simulink model "parallel_min_cost_function_vopt_6phase"  (R2022a)
settings: Solver=FixedStepDiscrete  StartTime=0.0  StopTime=10.0  RelTol=1e-3
undefined symbols (not defined in the file or in its folder): f_c
libraries: hdlsllib x18
settings Model: DataTypeOverride=Off  Creator=Andre Merx  LastModifiedBy=Andre Merx
settings SolverCC: AlgebraicLoopSolver=TrustRegion
settings DataIOCC: LimitDataPoints=on  SaveOutput=off  SaveTime=off
settings OptimizationCC: BlockReduction=off  ConditionallyExecuteInputs=off  DefaultParameterBehavior=Inlined  LifeSpan=inf
settings DebuggingCC: AlgebraicLoopMsg=error  SingleTaskRateTransMsg=error  UnconnectedInputMsg=warning  UnconnectedOutputMsg=warning  UnconnectedLineMsg=warning  AllowSymbolicDim=off  StrictBusMsg=ErrorOnBusTreatedAsVector  SFUnexpectedBacktrackingDiag=warning  SFNoUnconditionalDefaultTransitionDiag=warning  SFExecutionAtInitializationDiag=none  SFMachineParentedDataDiag=warning  ArithmeticOperatorsInVariantConditions=warning
settings HardwareCC: ProdBitPerPointer=32  ProdBitPerSizeT=32  ProdBitPerPtrDiffT=32  ProdLargestAtomicFloat=None  ProdIntDivRoundTo=Undefined  ProdEndianess=Unspecified  ProdWordSize=32  ProdHWDeviceType=ASIC/FPGA->ASIC/FPGA  ProdEqTarget=off
settings SFSimCC: SimUseLocalCustomCode=off  CustomCodeUndefinedFunction=UseInterfaceOnly
settings RTWCC: RTWUseLocalCustomCode=off
settings CodeAppCC: StateflowObjectComments=on
settings GRTTargetCC: TargetLangStandard=C89/C90 (ANSI)
settings ConfigComp: CovScope=ReferencedModels  CovMetricSettings=dw  CovSaveCumulativeToWorkspaceVar=on  CovSaveSingleToWorkspaceVar=on  CovExternalEMLEnable=off  CovSFcnEnable=off

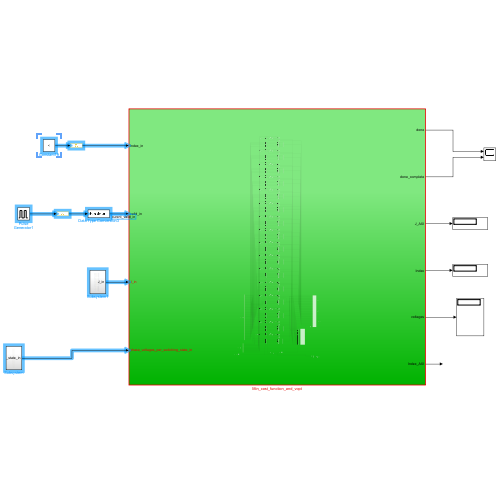
[thumbnail: Simulink's stored preview of the top-level diagram]
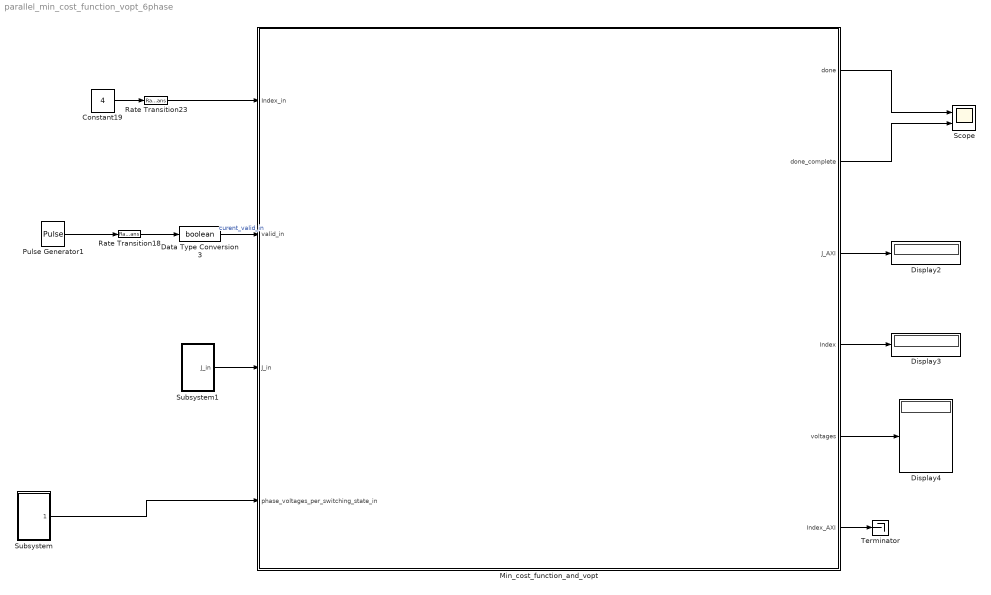
== system parallel_min_cost_function_vopt_6phase ==
  Constant19 : Constant  Value=4  OutDataTypeStr=int32  SampleTime=-1
  Data Type Conversion3 : DataTypeConversion  OutDataTypeStr=boolean  SaturateOnIntegerOverflow=off  RndMeth=Floor
  Display2 : Display
  Display3 : Display
  Display4 : Display
  Min_cost_function_and_vopt : Subsystem  TreatAsAtomicUnit=on
  Pulse Generator1 : DiscretePulseGenerator  PulseType=Time based  Period=1/f_c
  Rate Transition18 : RateTransition  OutPortSampleTime=Rt
  Rate Transition23 : RateTransition  OutPortSampleTime=Rt
  Scope : Scope  NumInputPorts=2
  Subsystem : Subsystem
  Subsystem1 : Subsystem
  Terminator : Terminator
  wires:
  Rate Transition23/1 -> Min_cost_function_and_vopt/1(Index_in)
  Constant19/1 -> Rate Transition23/1
  Rate Transition18/1 -> Data Type Conversion3/1
  Data Type Conversion3/1 -> Min_cost_function_and_vopt/2(valid_in)  "curent_valid_in"
  Pulse Generator1/1 -> Rate Transition18/1
  Subsystem1/1(J_in) -> Min_cost_function_and_vopt/3(J_in)
  Subsystem/1(phase_voltages_per_switching_state_in) -> Min_cost_function_and_vopt/4(phase_voltages_per_switching_state_in)
  Min_cost_function_and_vopt/1(done) -> Scope/1
  Min_cost_function_and_vopt/2(done_complete) -> Scope/2
  Min_cost_function_and_vopt/3(J_AXI) -> Display2/1
  Min_cost_function_and_vopt/4(Index) -> Display3/1
  Min_cost_function_and_vopt/5(voltages) -> Display4/1
  Min_cost_function_and_vopt/6(Index_AXI) -> Terminator/1

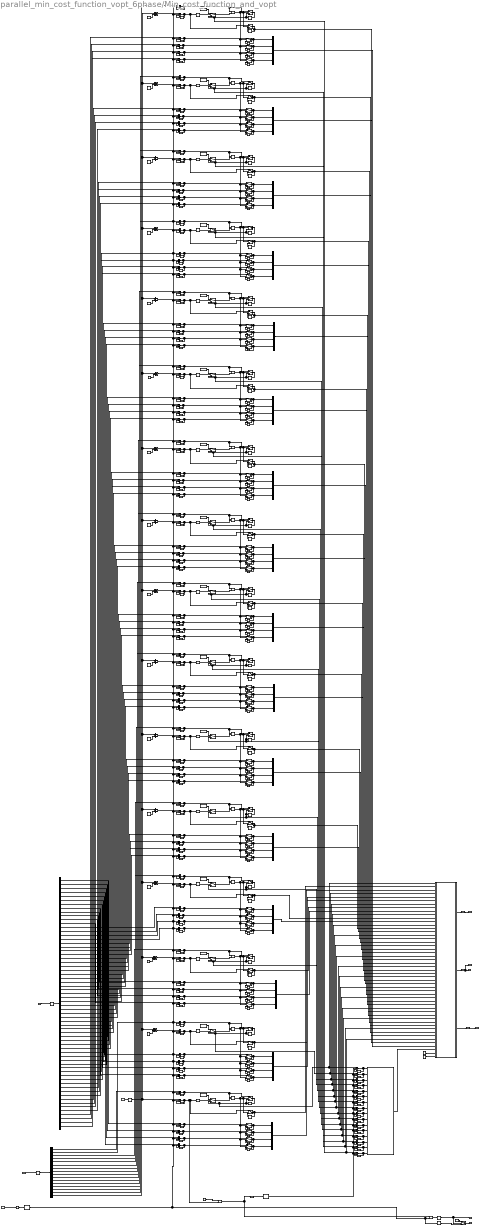
== system parallel_min_cost_function_vopt_6phase/Min_cost_function_and_vopt ==
  Index_in : Inport
  valid_in : Inport  Port=2
  J_in : Inport  Port=3
  phase_voltages_per_switching_state_in : Inport  Port=4
  Add{,1..14} (15 alike) : Sum
  Compare To Constant : hdlsllib/Logic and Bit Operations/Compare To Constant  relop=<=  const=1  OutDataTypeStr=boolean
      settings: SourceProductBaseCode=SL
  Compare To Constant1 : hdlsllib/Logic and Bit Operations/Compare To Constant  relop=<=  const=5  OutDataTypeStr=boolean
      settings: SourceProductBaseCode=SL
  Compare To Constant10 : hdlsllib/Logic and Bit Operations/Compare To Constant  relop=<=  const=41  OutDataTypeStr=boolean
      settings: SourceProductBaseCode=SL
  Compare To Constant11 : hdlsllib/Logic and Bit Operations/Compare To Constant  relop=<=  const=45  OutDataTypeStr=boolean
      settings: SourceProductBaseCode=SL
  Compare To Constant12 : hdlsllib/Logic and Bit Operations/Compare To Constant  relop=<=  const=49  OutDataTypeStr=boolean
      settings: SourceProductBaseCode=SL
  Compare To Constant13 : hdlsllib/Logic and Bit Operations/Compare To Constant  relop=<=  const=53  OutDataTypeStr=boolean
      settings: SourceProductBaseCode=SL
  Compare To Constant14 : hdlsllib/Logic and Bit Operations/Compare To Constant  relop=<=  const=57  OutDataTypeStr=boolean
      settings: SourceProductBaseCode=SL
  Compare To Constant15 : hdlsllib/Logic and Bit Operations/Compare To Constant  relop=<=  const=61  OutDataTypeStr=boolean
      settings: SourceProductBaseCode=SL
  Compare To Constant2 : hdlsllib/Logic and Bit Operations/Compare To Constant  relop=<=  const=9  OutDataTypeStr=boolean
      settings: SourceProductBaseCode=SL
  Compare To Constant3 : hdlsllib/Logic and Bit Operations/Compare To Constant  relop=<=  const=13  OutDataTypeStr=boolean
      settings: SourceProductBaseCode=SL
  Compare To Constant4 : hdlsllib/Logic and Bit Operations/Compare To Constant  relop=<=  const=17  OutDataTypeStr=boolean
      settings: SourceProductBaseCode=SL
  Compare To Constant5 : hdlsllib/Logic and Bit Operations/Compare To Constant  relop=<=  const=21  OutDataTypeStr=boolean
      settings: SourceProductBaseCode=SL
  Compare To Constant6 : hdlsllib/Logic and Bit Operations/Compare To Constant  relop=<=  const=25  OutDataTypeStr=boolean
      settings: SourceProductBaseCode=SL
  Compare To Constant7 : hdlsllib/Logic and Bit Operations/Compare To Constant  relop=<=  const=29  OutDataTypeStr=boolean
      settings: SourceProductBaseCode=SL
  Compare To Constant8 : hdlsllib/Logic and Bit Operations/Compare To Constant  relop=<=  const=33  OutDataTypeStr=boolean
      settings: SourceProductBaseCode=SL
  Compare To Constant9 : hdlsllib/Logic and Bit Operations/Compare To Constant  relop=<=  const=37  OutDataTypeStr=boolean
      settings: SourceProductBaseCode=SL
  Constant{,3..17} (16 alike) : Constant  Value=250  OutDataTypeStr=fixdt(1,20,11)  SampleTime=-1
  Constant1 : Constant  Value=4  OutDataTypeStr=int32  SampleTime=-1
  Constant18 : Constant  Value=4  OutDataTypeStr=int32  SampleTime=-1
  Constant19 : Constant  Value=8  OutDataTypeStr=int32  SampleTime=-1
  Constant2 : Constant  Value=0  OutDataTypeStr=boolean  SampleTime=-1
  Constant20 : Constant  Value=12  OutDataTypeStr=int32  SampleTime=-1
  Constant21 : Constant  Value=16  OutDataTypeStr=int32  SampleTime=-1
  Constant22 : Constant  Value=20  OutDataTypeStr=int32  SampleTime=-1
  Constant23 : Constant  Value=24  OutDataTypeStr=int32  SampleTime=-1
  Constant24 : Constant  Value=28  OutDataTypeStr=int32  SampleTime=-1
  Constant25 : Constant  Value=32  OutDataTypeStr=int32  SampleTime=-1
  Constant26 : Constant  Value=36  OutDataTypeStr=int32  SampleTime=-1
  Constant27 : Constant  Value=40  OutDataTypeStr=int32  SampleTime=-1
  Constant28 : Constant  Value=44  OutDataTypeStr=int32  SampleTime=-1
  Constant29 : Constant  Value=48  OutDataTypeStr=int32  SampleTime=-1
  Constant30 : Constant  Value=52  OutDataTypeStr=int32  SampleTime=-1
  Constant31 : Constant  Value=56  OutDataTypeStr=int32  SampleTime=-1
  Constant32 : Constant  Value=60  OutDataTypeStr=int32  SampleTime=-1
  Constant33 : Constant  Value=0  OutDataTypeStr=fixdt(1,20,11)  SampleTime=-1
  Constant34 : Constant  Value=[0;0;0;0]  OutDataTypeStr=fixdt(1,24,11)  SampleTime=-1
  Delay{,1..5,7..8,12..22,25..26,34..43,46,49..50,58..67,72..73,81..90,95..96,104..113,118..119,127..136,141..142,150..159,164..165,173..182,191..200,205..206,214..223,228..229,237..246,251..252,260..269,274..275,283..292,297..298,302..303,311..320,325..326,334..343,348..349,357..366,371..386} (216 alike) : Delay  DelayLength=1
  Delay23 : Delay  DelayLength=3
  Delay24 : Delay  DelayLength=3
  Demux : Demux  Outputs=16
  Demux1 : Demux  Outputs=64
  Detect Rise Positive : hdlsllib/Logic and Bit Operations/Detect Rise Positive  vinit=0  OutDataTypeStr=boolean
      settings: SourceProductBaseCode=SL
  Detect Rise Positive1 : hdlsllib/Logic and Bit Operations/Detect Rise Positive  vinit=0  OutDataTypeStr=boolean
      settings: SourceProductBaseCode=SL
  Logical Operator : Logic  AllPortsSameDT=off  OutDataTypeStr=boolean
  MATLAB Function : MATLAB Function  TreatAsAtomicUnit=on
  MinMax : MinMax  Inputs=16
  Mux{,1..15} (16 alike) : Mux
  Relational Operator{,2..16} (16 alike) : RelationalOperator  Operator=<=  OutDataTypeStr=boolean  RndMeth=Simplest  InputSameDT=off
  Relational Operator1 : RelationalOperator  Operator===  OutDataTypeStr=boolean  RndMeth=Simplest  InputSameDT=off
  Switch{,1,8..9,20..21,27..28,34..35,41..42,48..49,55..56,62..63,69..70,76..77,83..84,90..91,97..98,104..105,111..112} (32 alike) : Switch  Criteria=u2 > Threshold  OutDataTypeStr=fixdt(1,20,11)  SaturateOnIntegerOverflow=off  InputSameDT=off
  Switch{2,10,15,22,29,36,43,50,57,64,71,78,85,92,99,106} (16 alike) : Switch  Criteria=u2 > Threshold  OutDataTypeStr=int32  SaturateOnIntegerOverflow=off  InputSameDT=off
  Switch{3..6,11..14,16..19,23..26,30..33,37..40,44..47,51..54,58..61,65..68,72..75,79..82,86..89,93..96,100..103,107..110} (64 alike) : Switch  Criteria=u2 > Threshold  OutDataTypeStr=fixdt(1,24,11)  SaturateOnIntegerOverflow=off  InputSameDT=off
  Switch7 : Switch  Criteria=u2 > Threshold  SaturateOnIntegerOverflow=off  InputSameDT=off
  Switch_on{1,4,7,10,14,17,20,23,26,29,32,35,38,41,44,47,50,53,56,59,62,65,68,71,74,77,80,83,86,89,92,95,98..113} (48 alike) : Switch  Threshold=1  OutDataTypeStr=Inherit: Inherit via back propagation  RndMeth=Simplest  SaturateOnIntegerOverflow=off  InputSameDT=off
  Switch_on{2..3,5..6,8..9,11..12,15..16,18..19,21..22,24..25,27..28,30..31,33..34,36..37,39..40,42..43,45..46,48..49,51..52,54..55,57..58,60..61,63..64,66..67,69..70,72..73,75..76,78..79,81..82,84..85,87..88,90..91,93..94,96..97} (64 alike) : Switch  Threshold=1  OutDataTypeStr=fixdt(1,24,11)  RndMeth=Simplest  SaturateOnIntegerOverflow=off  InputSameDT=off
      Switch_on49 settings: LockScale=on
  done : Outport
  done_complete : Outport  Port=2
  J_AXI : Outport  Port=3
  Index : Outport  Port=4
  voltages : Outport  Port=5
  Index_AXI : Outport  Port=6
  wires:
  Demux/1 -> Switch_on4/1  "End_Cycle"
  Demux1/1 -> Switch_on2/1  "End_Cycle"
  Demux1/2 -> Switch_on3/1  "End_Cycle"
  Switch5/1 -> Mux/3, Delay4/1
  Delay3/1 -> Switch4/3
  Relational Operator/1 -> Switch5/2, Switch6/2, Switch4/2, Switch3/2, Switch2/2, Switch1/2
  Compare To Constant/1 -> Switch/2
  Switch1/1 -> Delay/1
  Switch6/1 -> Delay5/1, Mux/4
  Delay4/1 -> Switch5/3
  Switch4/1 -> Mux/2, Delay3/1
  Switch/1 -> Relational Operator/2
  Delay1/1 -> Switch2/3
  Delay5/1 -> Switch6/3
  Switch3/1 -> Mux/1, Delay2/1
  Delay2/1 -> Switch3/3
  Constant/1 -> Switch/1
  Switch_on4/1 -> Relational Operator/1, Switch1/1, Delay17/1
  Switch_on1/1 -> Delay18/1, Relational Operator1/2, Switch2/1, Compare To Constant/1
  Switch_on2/1 -> Delay19/1, Switch3/1
  Switch_on3/1 -> Delay20/1, Switch4/1
  Switch_on5/1 -> Switch5/1, Delay21/1
  Switch_on6/1 -> Switch6/1, Delay22/1
  Delay46/1 -> Detect Rise Positive/1
  valid_in/1 -> Delay46/1  "End_Cycle"
  Delay17/1 -> Switch_on4/3
  Delay8/1 -> Switch_on1/1, Add/1, Add3/1, Add7/1, Add10/1, Add12/1, Add14/1, Add13/1, Add11/1, Add9/1, Add8/1, Add6/1, Add5/1, Add4/1, Add2/1, Add1/1
  Delay18/1 -> Switch_on1/3
  Delay19/1 -> Switch_on2/3
  Delay20/1 -> Switch_on3/3
  Delay21/1 -> Switch_on5/3
  Delay22/1 -> Switch_on6/3
  Delay23/1 -> Switch7/2, done_complete/1
  Logical Operator/1 -> Delay23/1
  Delay24/1 -> Switch7/3
  Constant1/1 -> Relational Operator1/1
  Constant2/1 -> Switch7/1
  Switch7/1 -> done/1
  Demux1/3 -> Switch_on5/1  "End_Cycle"
  Demux1/4 -> Switch_on6/1  "End_Cycle"
  Demux/2 -> Switch_on10/1  "End_Cycle"
  Delay34/1 -> Switch_on10/3
  Switch8/1 -> Relational Operator2/2
  Switch_on8/1 -> Delay36/1, Switch11/1
  Demux1/6 -> Switch_on9/1  "End_Cycle"
  Delay26/1 -> Switch10/3
  Add/1 -> Switch_on7/1
  Delay36/1 -> Switch_on8/3
  Delay39/1 -> Switch_on11/3
  Switch_on7/1 -> Delay35/1, Switch10/1, Compare To Constant1/1
  Compare To Constant1/1 -> Switch8/2
  Switch_on9/1 -> Delay38/1, Switch12/1
  Delay40/1 -> Switch_on12/3
  Delay35/1 -> Switch_on7/3
  Switch_on11/1 -> Switch13/1, Delay39/1
  Delay43/1 -> Switch14/3
  Switch_on12/1 -> Switch14/1, Delay40/1
  Delay37/1 -> Switch11/3
  Relational Operator2/1 -> Switch13/2, Switch14/2, Switch12/2, Switch11/2, Switch10/2, Switch9/2
  Switch9/1 -> Delay25/1
  Delay42/1 -> Switch13/3
  Demux1/5 -> Switch_on8/1  "End_Cycle"
  Demux1/7 -> Switch_on11/1  "End_Cycle"
  Switch_on10/1 -> Relational Operator2/1, Switch9/1, Delay34/1
  Demux1/8 -> Switch_on12/1  "End_Cycle"
  Delay38/1 -> Switch_on9/3
  Constant3/1 -> Switch8/1
  Delay41/1 -> Switch12/3
  Delay61/1 -> Switch16/3
  Switch_on16/1 -> Switch19/1, Delay64/1
  Delay67/1 -> Switch19/3
  Switch_on15/1 -> Switch18/1, Delay63/1
  Delay59/1 -> Switch_on17/3
  Switch_on19/1 -> Delay62/1, Switch17/1
  Delay64/1 -> Switch_on16/3
  Switch_on17/1 -> Delay59/1, Switch15/1, Compare To Constant2/1
  Compare To Constant2/1 -> Switch20/2
  Demux1/10 -> Switch_on19/1  "End_Cycle"
  Delay50/1 -> Switch15/3
  Switch20/1 -> Relational Operator3/2
  Demux/3 -> Switch_on14/1  "End_Cycle"
  Delay65/1 -> Switch17/3
  Switch_on14/1 -> Relational Operator3/1, Switch21/1, Delay58/1
  Switch_on18/1 -> Delay60/1, Switch16/1
  Constant4/1 -> Switch20/1
  Demux1/11 -> Switch_on15/1  "End_Cycle"
  Delay63/1 -> Switch_on15/3
  Delay66/1 -> Switch18/3
  Switch21/1 -> Delay49/1
  Demux1/9 -> Switch_on18/1  "End_Cycle"
  Demux1/12 -> Switch_on16/1  "End_Cycle"
  Add1/1 -> Switch_on17/1
  Delay60/1 -> Switch_on18/3
  Relational Operator3/1 -> Switch18/2, Switch19/2, Switch17/2, Switch16/2, Switch15/2, Switch21/2
  Delay58/1 -> Switch_on14/3
  Delay62/1 -> Switch_on19/3
  Delay84/1 -> Switch23/3
  Switch_on22/1 -> Switch26/1, Delay87/1
  Delay90/1 -> Switch26/3
  Switch_on21/1 -> Switch25/1, Delay86/1
  Delay82/1 -> Switch_on23/3
  Switch_on25/1 -> Delay85/1, Switch24/1
  Delay87/1 -> Switch_on22/3
  Switch_on23/1 -> Delay82/1, Switch22/1, Compare To Constant3/1
  Compare To Constant3/1 -> Switch27/2
  Demux1/14 -> Switch_on25/1  "End_Cycle"
  Delay73/1 -> Switch22/3
  Switch27/1 -> Relational Operator4/2
  Demux/4 -> Switch_on20/1  "End_Cycle"
  Delay88/1 -> Switch24/3
  Switch_on20/1 -> Relational Operator4/1, Switch28/1, Delay81/1
  Switch_on24/1 -> Delay83/1, Switch23/1
  Constant5/1 -> Switch27/1
  Demux1/15 -> Switch_on21/1  "End_Cycle"
  Delay86/1 -> Switch_on21/3
  Delay89/1 -> Switch25/3
  Switch28/1 -> Delay72/1
  Demux1/13 -> Switch_on24/1  "End_Cycle"
  Demux1/16 -> Switch_on22/1  "End_Cycle"
  Add2/1 -> Switch_on23/1
  Delay83/1 -> Switch_on24/3
  Relational Operator4/1 -> Switch25/2, Switch26/2, Switch24/2, Switch23/2, Switch22/2, Switch28/2
  Delay81/1 -> Switch_on20/3
  Delay85/1 -> Switch_on25/3
  Delay107/1 -> Switch30/3
  Switch_on28/1 -> Switch33/1, Delay110/1
  Delay113/1 -> Switch33/3
  Switch_on27/1 -> Switch32/1, Delay109/1
  Delay105/1 -> Switch_on29/3
  Switch_on31/1 -> Delay108/1, Switch31/1
  Delay110/1 -> Switch_on28/3
  Switch_on29/1 -> Delay105/1, Switch29/1, Compare To Constant4/1
  Compare To Constant4/1 -> Switch34/2
  Demux1/18 -> Switch_on31/1  "End_Cycle"
  Delay96/1 -> Switch29/3
  Switch34/1 -> Relational Operator5/2
  Demux/5 -> Switch_on26/1  "End_Cycle"
  Delay111/1 -> Switch31/3
  Switch_on26/1 -> Relational Operator5/1, Switch35/1, Delay104/1
  Switch_on30/1 -> Delay106/1, Switch30/1
  Constant6/1 -> Switch34/1
  Demux1/19 -> Switch_on27/1  "End_Cycle"
  Delay109/1 -> Switch_on27/3
  Delay112/1 -> Switch32/3
  Switch35/1 -> Delay95/1
  Demux1/17 -> Switch_on30/1  "End_Cycle"
  Demux1/20 -> Switch_on28/1  "End_Cycle"
  Add3/1 -> Switch_on29/1
  Delay106/1 -> Switch_on30/3
  Relational Operator5/1 -> Switch32/2, Switch33/2, Switch31/2, Switch30/2, Switch29/2, Switch35/2
  Delay104/1 -> Switch_on26/3
  Delay108/1 -> Switch_on31/3
  Delay130/1 -> Switch37/3
  Switch_on34/1 -> Switch40/1, Delay133/1
  Delay136/1 -> Switch40/3
  Switch_on33/1 -> Switch39/1, Delay132/1
  Delay128/1 -> Switch_on35/3
  Switch_on37/1 -> Delay131/1, Switch38/1
  Delay133/1 -> Switch_on34/3
  Switch_on35/1 -> Delay128/1, Switch36/1, Compare To Constant5/1
  Compare To Constant5/1 -> Switch41/2
  Demux1/22 -> Switch_on37/1  "End_Cycle"
  Delay119/1 -> Switch36/3
  Switch41/1 -> Relational Operator6/2
  Demux/6 -> Switch_on32/1  "End_Cycle"
  Delay134/1 -> Switch38/3
  Switch_on32/1 -> Relational Operator6/1, Switch42/1, Delay127/1
  Switch_on36/1 -> Delay129/1, Switch37/1
  Constant7/1 -> Switch41/1
  Demux1/23 -> Switch_on33/1  "End_Cycle"
  Delay132/1 -> Switch_on33/3
  Delay135/1 -> Switch39/3
  Switch42/1 -> Delay118/1
  Demux1/21 -> Switch_on36/1  "End_Cycle"
  Demux1/24 -> Switch_on34/1  "End_Cycle"
  Add4/1 -> Switch_on35/1
  Delay129/1 -> Switch_on36/3
  Relational Operator6/1 -> Switch39/2, Switch40/2, Switch38/2, Switch37/2, Switch36/2, Switch42/2
  Delay127/1 -> Switch_on32/3
  Delay131/1 -> Switch_on37/3
  Delay153/1 -> Switch44/3
  Switch_on40/1 -> Switch47/1, Delay156/1
  Delay159/1 -> Switch47/3
  Switch_on39/1 -> Switch46/1, Delay155/1
  Delay151/1 -> Switch_on41/3
  Switch_on43/1 -> Delay154/1, Switch45/1
  Delay156/1 -> Switch_on40/3
  Switch_on41/1 -> Delay151/1, Switch43/1, Compare To Constant6/1
  Compare To Constant6/1 -> Switch48/2
  Demux1/26 -> Switch_on43/1  "End_Cycle"
  Delay142/1 -> Switch43/3
  Switch48/1 -> Relational Operator7/2
  Delay157/1 -> Switch45/3
  Switch_on38/1 -> Relational Operator7/1, Switch49/1, Delay150/1
  Switch_on42/1 -> Delay152/1, Switch44/1
  Constant8/1 -> Switch48/1
  Demux1/27 -> Switch_on39/1  "End_Cycle"
  Delay155/1 -> Switch_on39/3
  Delay158/1 -> Switch46/3
  Switch49/1 -> Delay141/1
  Demux1/25 -> Switch_on42/1  "End_Cycle"
  Demux1/28 -> Switch_on40/1  "End_Cycle"
  Add5/1 -> Switch_on41/1
  Delay152/1 -> Switch_on42/3
  Relational Operator7/1 -> Switch46/2, Switch47/2, Switch45/2, Switch44/2, Switch43/2, Switch49/2
  Delay150/1 -> Switch_on38/3
  Delay154/1 -> Switch_on43/3
  Delay176/1 -> Switch51/3
  Switch_on46/1 -> Switch54/1, Delay179/1
  Delay182/1 -> Switch54/3
  Switch_on45/1 -> Switch53/1, Delay178/1
  Delay174/1 -> Switch_on47/3
  Switch_on49/1 -> Delay177/1, Switch52/1
  Delay179/1 -> Switch_on46/3
  Switch_on47/1 -> Delay174/1, Switch50/1, Compare To Constant7/1
  Compare To Constant7/1 -> Switch55/2
  Demux1/30 -> Switch_on49/1  "End_Cycle"
  Delay165/1 -> Switch50/3
  Switch55/1 -> Relational Operator8/2
  Demux/8 -> Switch_on44/1  "End_Cycle"
  Delay180/1 -> Switch52/3
  Switch_on44/1 -> Relational Operator8/1, Switch56/1, Delay173/1
  Switch_on48/1 -> Delay175/1, Switch51/1
  Constant9/1 -> Switch55/1
  Demux1/31 -> Switch_on45/1  "End_Cycle"
  Delay178/1 -> Switch_on45/3
  Delay181/1 -> Switch53/3
  Switch56/1 -> Delay164/1
  Demux1/29 -> Switch_on48/1  "End_Cycle"
  Demux1/32 -> Switch_on46/1  "End_Cycle"
  Add6/1 -> Switch_on47/1
  Delay175/1 -> Switch_on48/3
  Relational Operator8/1 -> Switch53/2, Switch54/2, Switch52/2, Switch51/2, Switch50/2, Switch56/2
  Delay173/1 -> Switch_on44/3
  Delay177/1 -> Switch_on49/3
  Delay264/1 -> Switch_on79/3
  Relational Operator13/1 -> Switch88/2, Switch89/2, Switch87/2, Switch86/2, Switch85/2, Switch91/2
  Add11/1 -> Switch_on77/1
  Demux1/49 -> Switch_on78/1  "End_Cycle"
  Demux1/51 -> Switch_on75/1  "End_Cycle"
  Delay268/1 -> Switch88/3
  Constant14/1 -> Switch90/1
  Delay252/1 -> Switch85/3
  Compare To Constant12/1 -> Switch90/2
  Switch_on75/1 -> Switch88/1, Delay265/1
  Delay291/1 -> Switch60/3
  Demux1/35 -> Switch_on51/1  "End_Cycle"
  Switch_on74/1 -> Relational Operator13/1, Switch91/1, Delay260/1
  Demux/13 -> Switch_on74/1  "End_Cycle"
  Switch_on54/1 -> Delay285/1, Switch58/1
  Delay290/1 -> Switch59/3
  Relational Operator9/1 -> Switch60/2, Switch61/2, Switch59/2, Switch58/2, Switch57/2, Switch63/2
  Switch90/1 -> Relational Operator13/2
  Delay285/1 -> Switch_on54/3
  Switch_on55/1 -> Delay287/1, Switch59/1
  Delay284/1 -> Switch_on53/3
  Delay292/1 -> Switch61/3
  Switch_on52/1 -> Switch61/1, Delay289/1
  Switch62/1 -> Relational Operator9/2
  Demux/9 -> Switch_on50/1  "End_Cycle"
  Demux1/34 -> Switch_on55/1  "End_Cycle"
  Compare To Constant8/1 -> Switch62/2
  Switch_on53/1 -> Delay284/1, Switch57/1, Compare To Constant8/1
  Delay192/1 -> Switch_on59/3
  Switch_on57/1 -> Switch67/1, Delay196/1
  Switch_on58/1 -> Switch68/1, Delay197/1
  Demux1/52 -> Switch_on76/1  "End_Cycle"
  Compare To Constant11/1 -> Switch83/2
  Constant10/1 -> Switch62/1
  Switch_on73/1 -> Delay241/1, Switch80/1
  Delay262/1 -> Switch_on78/3
  Switch_on69/1 -> Switch81/1, Delay242/1
  Delay246/1 -> Switch82/3
  Delay266/1 -> Switch_on76/3
  Delay263/1 -> Switch86/3
  Switch_on70/1 -> Switch82/1, Delay243/1
  Delay240/1 -> Switch79/3
  Demux1/40 -> Switch_on58/1  "End_Cycle"
  Switch70/1 -> Delay297/1
  Delay199/1 -> Switch67/3
  Delay194/1 -> Switch65/3
  Demux1/33 -> Switch_on54/1  "End_Cycle"
  Demux1/39 -> Switch_on57/1  "End_Cycle"
  Delay196/1 -> Switch_on57/3
  Constant11/1 -> Switch69/1
  Switch_on78/1 -> Delay262/1, Switch86/1
  Switch_on60/1 -> Delay193/1, Switch65/1
  Delay298/1 -> Switch64/3
  Demux/10 -> Switch_on56/1  "End_Cycle"
  Demux1/38 -> Switch_on61/1  "End_Cycle"
  Switch_on56/1 -> Relational Operator10/1, Switch70/1, Delay191/1
  Switch_on79/1 -> Delay264/1, Switch87/1
  Delay198/1 -> Switch66/3
  Demux1/50 -> Switch_on79/1  "End_Cycle"
  Delay269/1 -> Switch89/3
  Delay197/1 -> Switch_on58/3
  Switch_on59/1 -> Delay192/1, Switch64/1, Compare To Constant9/1
  Delay243/1 -> Switch_on70/3
  Delay286/1 -> Switch58/3
  Switch_on76/1 -> Switch89/1, Delay266/1
  Delay287/1 -> Switch_on55/3
  Delay289/1 -> Switch_on52/3
  Switch_on51/1 -> Switch60/1, Delay288/1
  Delay239/1 -> Switch_on72/3
  Delay275/1 -> Switch57/3
  Add10/1 -> Switch_on71/1
  Relational Operator12/1 -> Switch81/2, Switch82/2, Switch80/2, Switch79/2, Switch78/2, Switch84/2
  Demux1/48 -> Switch_on70/1  "End_Cycle"
  Demux1/45 -> Switch_on72/1  "End_Cycle"
  Switch84/1 -> Delay228/1
  Demux1/47 -> Switch_on69/1  "End_Cycle"
  Constant13/1 -> Switch83/1
  Switch_on72/1 -> Delay239/1, Switch79/1
  Delay267/1 -> Switch87/3
  Switch_on68/1 -> Relational Operator12/1, Switch84/1, Delay237/1
  Switch83/1 -> Relational Operator12/2
  Demux1/37 -> Switch_on60/1  "End_Cycle"
  Delay229/1 -> Switch78/3
  Delay195/1 -> Switch_on61/3
  Switch69/1 -> Relational Operator10/2
  Delay217/1 -> Switch72/3
  Delay265/1 -> Switch_on75/3
  Demux1/46 -> Switch_on73/1  "End_Cycle"
  Switch_on63/1 -> Switch74/1, Delay219/1
  Switch_on64/1 -> Switch75/1, Delay220/1
  Delay244/1 -> Switch80/3
  Switch_on71/1 -> Delay238/1, Switch78/1, Compare To Constant11/1
  Delay220/1 -> Switch_on64/3
  Delay223/1 -> Switch75/3
  Switch_on61/1 -> Delay195/1, Switch66/1
  Demux1/36 -> Switch_on52/1  "End_Cycle"
  Switch_on67/1 -> Delay218/1, Switch73/1
  Delay218/1 -> Switch_on67/3
  Delay193/1 -> Switch_on60/3
  Delay191/1 -> Switch_on56/3
  Switch63/1 -> Delay274/1
  Delay261/1 -> Switch_on77/3
  Relational Operator11/1 -> Switch74/2, Switch75/2, Switch73/2, Switch72/2, Switch71/2, Switch77/2
  Delay214/1 -> Switch_on62/3
  Delay242/1 -> Switch_on69/3
  Delay216/1 -> Switch_on66/3
  Add9/1 -> Switch_on65/1
  Switch77/1 -> Delay205/1
  Switch_on50/1 -> Relational Operator9/1, Switch63/1, Delay283/1
  Delay200/1 -> Switch68/3
  Delay222/1 -> Switch74/3
  Delay219/1 -> Switch_on63/3
  Delay288/1 -> Switch_on51/3
  Demux1/43 -> Switch_on63/1  "End_Cycle"
  Add8/1 -> Switch_on59/1
  Switch_on66/1 -> Delay216/1, Switch72/1
  Demux1/44 -> Switch_on64/1  "End_Cycle"
  Delay260/1 -> Switch_on74/3
  Compare To Constant9/1 -> Switch69/2
  Constant12/1 -> Switch76/1
  Delay245/1 -> Switch81/3
  Demux/11 -> Switch_on62/1  "End_Cycle"
  Delay206/1 -> Switch71/3
  Delay215/1 -> Switch_on65/3
  Delay221/1 -> Switch73/3
  Demux/12 -> Switch_on68/1  "End_Cycle"
  Add7/1 -> Switch_on53/1
  Switch76/1 -> Relational Operator11/2
  Delay241/1 -> Switch_on73/3
  Delay238/1 -> Switch_on71/3
  Relational Operator10/1 -> Switch67/2, Switch68/2, Switch66/2, Switch65/2, Switch64/2, Switch70/2
  Compare To Constant10/1 -> Switch76/2
  Switch_on65/1 -> Delay215/1, Switch71/1, Compare To Constant10/1
  Switch_on77/1 -> Delay261/1, Switch85/1, Compare To Constant12/1
  Delay283/1 -> Switch_on50/3
  Delay237/1 -> Switch_on68/3
  Demux1/41 -> Switch_on66/1  "End_Cycle"
  Switch_on62/1 -> Relational Operator11/1, Switch77/1, Delay214/1
  Demux1/42 -> Switch_on67/1  "End_Cycle"
  Switch91/1 -> Delay251/1
  Switch_on83/1 -> Delay312/1, Switch92/1, Compare To Constant13/1
  Switch112/1 -> Delay348/1
  Compare To Constant13/1 -> Switch97/2
  Delay335/1 -> Switch_on89/3
  Demux1/53 -> Switch_on84/1  "End_Cycle"
  Switch97/1 -> Relational Operator14/2
  Delay318/1 -> Switch94/3
  Delay303/1 -> Switch92/3
  Demux/15 -> Switch_on86/1  "End_Cycle"
  Delay312/1 -> Switch_on83/3
  Constant15/1 -> Switch97/1
  Delay342/1 -> Switch102/3
  Demux/14 -> Switch_on80/1  "End_Cycle"
  Demux1/56 -> Switch_on82/1  "End_Cycle"
  Delay319/1 -> Switch95/3
  Switch98/1 -> Delay302/1
  Demux/16 -> Switch_on92/1  "End_Cycle"
  Switch_on92/1 -> Relational Operator16/1, Switch112/1, Delay357/1
  Constant17/1 -> Switch111/1
  Delay357/1 -> Switch_on92/3
  Delay349/1 -> Switch106/3
  Delay365/1 -> Switch109/3
  Add14/1 -> Switch_on95/1
  Demux1/63 -> Switch_on93/1  "End_Cycle"
  Switch_on84/1 -> Delay313/1, Switch93/1
  Delay316/1 -> Switch_on81/3
  Relational Operator14/1 -> Switch95/2, Switch96/2, Switch94/2, Switch93/2, Switch92/2, Switch98/2
  Delay334/1 -> Switch_on86/3
  Delay358/1 -> Switch_on95/3
  Delay339/1 -> Switch_on87/3
  Demux1/54 -> Switch_on85/1  "End_Cycle"
  Delay311/1 -> Switch_on80/3
  Switch_on85/1 -> Delay315/1, Switch94/1
  Switch111/1 -> Relational Operator16/2
  Switch_on81/1 -> Switch95/1, Delay316/1
  Delay317/1 -> Switch_on82/3
  Switch_on93/1 -> Switch109/1, Delay362/1
  Switch_on89/1 -> Delay335/1, Switch99/1, Compare To Constant14/1
  Switch_on82/1 -> Switch96/1, Delay317/1
  Delay362/1 -> Switch_on93/3
  Delay314/1 -> Switch93/3
  Demux1/58 -> Switch_on91/1  "End_Cycle"
  Switch104/1 -> Relational Operator15/2
  Switch_on95/1 -> Delay358/1, Switch106/1, Compare To Constant15/1
  Delay315/1 -> Switch_on85/3
  Switch_on86/1 -> Relational Operator15/1, Switch105/1, Delay334/1
  Delay326/1 -> Switch99/3
  Constant16/1 -> Switch104/1
  Switch_on90/1 -> Delay336/1, Switch100/1
  Demux1/60 -> Switch_on88/1  "End_Cycle"
  Relational Operator15/1 -> Switch102/2, Switch103/2, Switch101/2, Switch100/2, Switch99/2, Switch105/2
  Delay361/1 -> Switch_on97/3
  Switch105/1 -> Delay325/1
  Delay341/1 -> Switch101/3
  Compare To Constant15/1 -> Switch111/2
  Add13/1 -> Switch_on89/1
  Switch_on94/1 -> Switch110/1, Delay363/1
  Delay313/1 -> Switch_on84/3
  Delay340/1 -> Switch_on88/3
  Delay366/1 -> Switch110/3
  Demux1/62 -> Switch_on97/1  "End_Cycle"
  Delay320/1 -> Switch96/3
  Switch_on80/1 -> Relational Operator14/1, Switch98/1, Delay311/1
  Relational Operator16/1 -> Switch109/2, Switch110/2, Switch108/2, Switch107/2, Switch106/2, Switch112/2
  Detect Rise Positive/1 -> Delay24/1, Logical Operator/2, Switch_on92/2, Switch_on95/2, Switch_on96/2, Switch_on97/2, Switch_on93/2, Switch_on94/2, Switch_on86/2, Switch_on89/2, Switch_on90/2, Switch_on91/2, Switch_on87/2, Switch_on88/2, Switch_on80/2, Switch_on83/2, Switch_on84/2, Switch_on85/2, Switch_on81/2, Switch_on82/2, Switch_on74/2, Switch_on77/2, Switch_on78/2, Switch_on79/2, Switch_on75/2, Switch_on76/2, Switch_on68/2, Switch_on71/2, Switch_on72/2, Switch_on73/2, Switch_on69/2, Switch_on70/2, Switch_on62/2, Switch_on65/2, Switch_on66/2, Switch_on67/2, Switch_on63/2, Switch_on64/2, Switch_on56/2, Switch_on59/2, Switch_on60/2, Switch_on61/2, Switch_on57/2, Switch_on58/2, Switch_on50/2, Switch_on53/2, Switch_on54/2, Switch_on55/2, Switch_on51/2, Switch_on52/2, Switch_on44/2, Switch_on47/2, Switch_on48/2, Switch_on49/2, Switch_on45/2, Switch_on46/2, Switch_on38/2, Switch_on41/2, Switch_on42/2, Switch_on43/2, Switch_on39/2, Switch_on40/2, Switch_on32/2, Switch_on35/2, Switch_on36/2, Switch_on37/2, Switch_on33/2, Switch_on34/2, Switch_on26/2, Switch_on29/2, Switch_on30/2, Switch_on31/2, Switch_on27/2, Switch_on28/2, Switch_on20/2, Switch_on23/2, Switch_on24/2, Switch_on25/2, Switch_on21/2, Switch_on22/2, Switch_on14/2, Switch_on17/2, Switch_on18/2, Switch_on19/2, Switch_on15/2, Switch_on16/2, Switch_on10/2, Switch_on7/2, Switch_on8/2, Switch_on9/2, Switch_on11/2, Switch_on12/2, Switch_on4/2, Switch_on1/2, Switch_on2/2, Switch_on3/2, Switch_on5/2, Switch_on6/2  "End_Cycle"
  Delay336/1 -> Switch_on90/3
  Demux1/61 -> Switch_on96/1  "End_Cycle"
  Switch_on96/1 -> Delay359/1, Switch107/1
  Delay360/1 -> Switch107/3
  Switch_on91/1 -> Delay338/1, Switch101/1
  Demux1/57 -> Switch_on90/1  "End_Cycle"
  Delay338/1 -> Switch_on91/3
  Switch_on87/1 -> Switch102/1, Delay339/1
  Demux1/55 -> Switch_on81/1  "End_Cycle"
  Switch_on97/1 -> Delay361/1, Switch108/1
  Delay363/1 -> Switch_on94/3
  Delay359/1 -> Switch_on96/3
  Delay337/1 -> Switch100/3
  Delay364/1 -> Switch108/3
  Switch_on88/1 -> Switch103/1, Delay340/1
  Demux1/64 -> Switch_on94/1  "End_Cycle"
  Demux1/59 -> Switch_on87/1  "End_Cycle"
  Add12/1 -> Switch_on83/1
  Delay343/1 -> Switch103/3
  Compare To Constant14/1 -> Switch104/2
  Constant18/1 -> Add/2
  Constant19/1 -> Add1/2
  Constant20/1 -> Add2/2
  Constant21/1 -> Add3/2
  Constant22/1 -> Add4/2
  Constant23/1 -> Add5/2
  Constant24/1 -> Add6/2
  Constant25/1 -> Add7/2
  Constant26/1 -> Add8/2
  Constant27/1 -> Add9/2
  Constant28/1 -> Add10/2
  Constant29/1 -> Add11/2
  Constant30/1 -> Add12/2
  Constant31/1 -> Add13/2
  Constant32/1 -> Add14/2
  Index_in/1 -> Delay8/1
  Delay371/1 -> Switch_on98/3
  Switch_on98/1 -> Delay371/1, MinMax/1
  Switch_on99/1 -> MinMax/2, Delay372/1
  Delay372/1 -> Switch_on99/3
  Switch_on100/1 -> MinMax/3, Delay373/1
  Delay373/1 -> Switch_on100/3
  Switch_on101/1 -> MinMax/4, Delay374/1
  Delay374/1 -> Switch_on101/3
  Delay376/1 -> Switch_on105/3
  Switch_on102/1 -> MinMax/7, Delay377/1
  Delay377/1 -> Switch_on102/3
  Delay141/1 -> MATLAB Function/19(J_7), Switch_on102/1, Switch48/3, Switch49/3
  Switch_on104/1 -> MinMax/5, Delay375/1
  Delay375/1 -> Switch_on104/3
  Switch_on105/1 -> MinMax/6, Delay376/1
  Switch_on103/1 -> MinMax/8, Delay378/1
  Delay378/1 -> Switch_on103/3
  Delay380/1 -> Switch_on109/3
  Switch_on106/1 -> MinMax/11, Delay381/1
  Delay381/1 -> Switch_on106/3
  Switch_on108/1 -> MinMax/9, Delay379/1
  Delay379/1 -> Switch_on108/3
  Switch_on109/1 -> MinMax/10, Delay380/1
  Switch_on107/1 -> MinMax/12, Delay382/1
  Delay382/1 -> Switch_on107/3
  Delay384/1 -> Switch_on113/3
  Switch_on110/1 -> MinMax/15, Delay385/1
  Delay385/1 -> Switch_on110/3
  Relational Operator1/1 -> Logical Operator/1, Delay15/1  "End_Cycle"
  Switch_on112/1 -> MinMax/13, Delay383/1
  Delay383/1 -> Switch_on112/3
  Switch_on113/1 -> MinMax/14, Delay384/1
  Switch_on111/1 -> MinMax/16, Delay386/1
  Delay386/1 -> Switch_on111/3
  Detect Rise Positive1/1 -> Switch_on98/2, Switch_on99/2, Switch_on100/2, Switch_on101/2, Switch_on104/2, Switch_on105/2, Switch_on102/2, Switch_on103/2, Switch_on108/2, Switch_on109/2, Switch_on106/2, Switch_on107/2, Switch_on112/2, Switch_on113/2, Switch_on110/2, Switch_on111/2  "End_Cycle"
  MinMax/1 -> MATLAB Function/49(min)
  Delay/1 -> MATLAB Function/1(J_1), Switch_on98/1, Switch/3, Switch1/3
  Delay25/1 -> Switch_on99/1, MATLAB Function/4(J_2), Switch8/3, Switch9/3
  Delay49/1 -> Switch_on100/1, MATLAB Function/7(J_3), Switch20/3, Switch21/3
  Delay72/1 -> Switch_on101/1, MATLAB Function/10(J_4), Switch27/3, Switch28/3
  Delay95/1 -> Switch34/3, Switch_on104/1, MATLAB Function/13(J_5), Switch35/3
  Delay118/1 -> Switch41/3, MATLAB Function/16(J_6), Switch_on105/1, Switch42/3
  Delay164/1 -> MATLAB Function/22(J_8), Switch_on103/1, Switch55/3, Switch56/3
  Delay274/1 -> MATLAB Function/25(J_9), Switch_on108/1, Switch62/3, Switch63/3
  Delay297/1 -> MATLAB Function/28(J_10), Switch_on109/1, Switch69/3, Switch70/3
  Delay205/1 -> MATLAB Function/31(J_11), Switch_on106/1, Switch76/3, Switch77/3
  Delay228/1 -> MATLAB Function/34(J_12), Switch_on107/1, Switch83/3, Switch84/3
  Delay251/1 -> MATLAB Function/37(J_13), Switch_on112/1, Switch90/3, Switch91/3
  Delay302/1 -> MATLAB Function/40(J_14), Switch_on113/1, Switch97/3, Switch98/3
  Delay325/1 -> MATLAB Function/43(J_15), Switch_on110/1, Switch104/3, Switch105/3
  Delay348/1 -> MATLAB Function/46(J_16), Switch_on111/1, Switch111/3, Switch112/3
  Switch2/1 -> MATLAB Function/2(Index_1), Delay1/1
  Switch10/1 -> MATLAB Function/5(Index_2), Delay26/1
  Switch15/1 -> MATLAB Function/8(Index_3), Delay50/1
  Switch22/1 -> MATLAB Function/11(Index_4), Delay73/1
  Switch29/1 -> MATLAB Function/14(Index_5), Delay96/1
  Switch36/1 -> MATLAB Function/17(Index_6), Delay119/1
  Switch43/1 -> MATLAB Function/20(Index_7), Delay142/1
  Switch50/1 -> MATLAB Function/23(Index_8), Delay165/1
  Switch57/1 -> MATLAB Function/26(Index_9), Delay275/1
  Switch71/1 -> MATLAB Function/32(Index_11), Delay206/1
  Switch78/1 -> MATLAB Function/35(Index_12), Delay229/1
  Switch85/1 -> MATLAB Function/38(Index_13), Delay252/1
  Switch92/1 -> MATLAB Function/41(Index_14), Delay303/1
  Switch99/1 -> MATLAB Function/44(Index_15), Delay326/1
  Switch106/1 -> MATLAB Function/47(Index_16), Delay349/1
  Switch64/1 -> MATLAB Function/29(Index_10), Delay298/1
  Switch13/1 -> Mux1/3, Delay42/1
  Switch12/1 -> Mux1/2, Delay41/1
  Switch14/1 -> Mux1/4, Delay43/1
  Switch11/1 -> Mux1/1, Delay37/1
  Switch18/1 -> Mux2/3, Delay66/1
  Switch17/1 -> Mux2/2, Delay65/1
  Switch19/1 -> Mux2/4, Delay67/1
  Switch16/1 -> Mux2/1, Delay61/1
  Switch25/1 -> Delay89/1, Mux3/3
  Switch24/1 -> Mux3/2, Delay88/1
  Switch26/1 -> Mux3/4, Delay90/1
  Switch23/1 -> Mux3/1, Delay84/1
  Switch32/1 -> Mux4/3, Delay112/1
  Switch31/1 -> Mux4/2, Delay111/1
  Switch33/1 -> Mux4/4, Delay113/1
  Switch30/1 -> Delay107/1, Mux4/1
  Switch39/1 -> Mux5/3, Delay135/1
  Switch38/1 -> Delay134/1, Mux5/2
  Switch40/1 -> Mux5/4, Delay136/1
  Switch37/1 -> Mux5/1, Delay130/1
  Switch46/1 -> Mux6/3, Delay158/1
  Switch45/1 -> Mux6/2, Delay157/1
  Switch47/1 -> Mux6/4, Delay159/1
  Switch44/1 -> Mux6/1, Delay153/1
  Switch53/1 -> Mux7/3, Delay181/1
  Switch52/1 -> Mux7/2, Delay180/1
  Switch54/1 -> Mux7/4, Delay182/1
  Switch51/1 -> Mux7/1, Delay176/1
  Switch60/1 -> Mux8/3, Delay291/1
  Switch59/1 -> Delay290/1, Mux8/2
  Switch61/1 -> Mux8/4, Delay292/1
  Switch58/1 -> Delay286/1, Mux8/1
  Switch67/1 -> Mux9/3, Delay199/1
  Switch66/1 -> Mux9/2, Delay198/1
  Switch68/1 -> Mux9/4, Delay200/1
  Switch65/1 -> Mux9/1, Delay194/1
  Switch74/1 -> Mux10/3, Delay222/1
  Switch73/1 -> Mux10/2, Delay221/1
  Switch75/1 -> Mux10/4, Delay223/1
  Switch72/1 -> Mux10/1, Delay217/1
  Switch88/1 -> Mux12/3, Delay268/1
  Switch87/1 -> Mux12/2, Delay267/1
  Switch89/1 -> Mux12/4, Delay269/1
  Switch86/1 -> Mux12/1, Delay263/1
  Switch95/1 -> Mux13/3, Delay319/1
  Switch94/1 -> Mux13/2, Delay318/1
  Switch96/1 -> Mux13/4, Delay320/1
  Switch93/1 -> Mux13/1, Delay314/1
  Switch102/1 -> Mux14/3, Delay342/1
  Switch101/1 -> Mux14/2, Delay341/1
  Switch103/1 -> Mux14/4, Delay343/1
  Switch100/1 -> Mux14/1, Delay337/1
  Switch109/1 -> Mux15/3, Delay365/1
  Switch108/1 -> Mux15/2, Delay364/1
  Switch110/1 -> Mux15/4, Delay366/1
  Switch107/1 -> Mux15/1, Delay360/1
  Mux/1 -> MATLAB Function/3(voltages_1)
  Mux1/1 -> MATLAB Function/6(voltages_2)
  Mux2/1 -> MATLAB Function/9(voltages_3)
  Mux3/1 -> MATLAB Function/12(voltages_4)
  Mux4/1 -> MATLAB Function/15(voltages_5)
  Mux5/1 -> MATLAB Function/18(voltages_6)
  Mux6/1 -> MATLAB Function/21(voltages_7)
  Mux7/1 -> MATLAB Function/24(voltages_8)
  Mux8/1 -> MATLAB Function/27(voltages_9)
  Mux9/1 -> MATLAB Function/30(voltages_10)
  Mux10/1 -> MATLAB Function/33(voltages_11)
  Mux11/1 -> MATLAB Function/36(voltages_12)
  Mux12/1 -> MATLAB Function/39(voltages_13)
  Mux13/1 -> MATLAB Function/42(voltages_14)
  Mux14/1 -> MATLAB Function/45(voltages_15)
  Mux15/1 -> MATLAB Function/48(voltages_16)
  MATLAB Function/1(J) -> Delay12/1
  MATLAB Function/2(Index) -> Delay13/1
  MATLAB Function/3(voltages) -> Delay14/1
  Delay12/1 -> J_AXI/1
  Delay13/1 -> Index_AXI/1, Index/1
  Delay14/1 -> voltages/1
  Switch80/1 -> Delay244/1, Mux11/2
  Switch79/1 -> Mux11/1, Delay240/1
  Switch82/1 -> Mux11/4, Delay246/1
  Switch81/1 -> Mux11/3, Delay245/1
  Constant33/1 -> MATLAB Function/50(J_default)
  Constant34/1 -> MATLAB Function/51(voltages_default)
  Delay15/1 -> Detect Rise Positive1/1
  Demux/7 -> Switch_on38/1  "End_Cycle"
  J_in/1 -> Delay7/1  "End_Cycle"
  phase_voltages_per_switching_state_in/1 -> Delay16/1  "End_Cycle"
  Delay16/1 -> Demux1/1
  Delay7/1 -> Demux/1

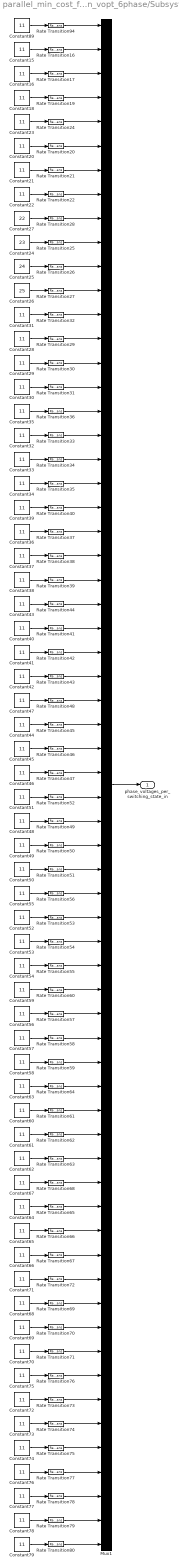
== system parallel_min_cost_function_vopt_6phase/Subsystem ==
  Constant{15..16,18,20..23,28..79,89} (60 alike) : Constant  Value=11  OutDataTypeStr=fixdt(1,24,11)  SampleTime=-1  LockScale=on
  Constant24 : Constant  Value=23  OutDataTypeStr=fixdt(1,24,11)  SampleTime=-1  LockScale=on
  Constant25 : Constant  Value=24  OutDataTypeStr=fixdt(1,24,11)  SampleTime=-1  LockScale=on
  Constant26 : Constant  Value=25  OutDataTypeStr=fixdt(1,24,11)  SampleTime=-1  LockScale=on
  Constant27 : Constant  Value=22  OutDataTypeStr=fixdt(1,24,11)  SampleTime=-1  LockScale=on
  Mux1 : Mux  Inputs=64
  Rate Transition{16..17,19..22,24..80,94} (64 alike) : RateTransition  OutPortSampleTime=Rt
  phase_voltages_per_switching_state_in : Outport  VectorParamsAs1DForOutWhenUnconnected=off
  wires:
  Rate Transition54/1 -> Mux1/39
  Rate Transition36/1 -> Mux1/17
  Constant56/1 -> Rate Transition57/1
  Rate Transition78/1 -> Mux1/62
  Constant35/1 -> Rate Transition36/1
  Constant61/1 -> Rate Transition62/1
  Constant42/1 -> Rate Transition43/1
  Mux1/1 -> phase_voltages_per_switching_state_in/1
  Constant48/1 -> Rate Transition49/1
  Constant24/1 -> Rate Transition25/1
  Constant32/1 -> Rate Transition33/1
  Rate Transition59/1 -> Mux1/44
  Rate Transition62/1 -> Mux1/47
  Rate Transition52/1 -> Mux1/33
  Constant18/1 -> Rate Transition19/1
  Rate Transition94/1 -> Mux1/1
  Constant36/1 -> Rate Transition37/1
  Rate Transition34/1 -> Mux1/19
  Constant75/1 -> Rate Transition76/1
  Constant37/1 -> Rate Transition38/1
  Rate Transition48/1 -> Mux1/29
  Rate Transition73/1 -> Mux1/58
  Rate Transition71/1 -> Mux1/56
  Rate Transition80/1 -> Mux1/64
  Constant43/1 -> Rate Transition44/1
  Constant20/1 -> Rate Transition20/1
  Constant70/1 -> Rate Transition71/1
  Rate Transition77/1 -> Mux1/61
  Rate Transition28/1 -> Mux1/9
  Constant66/1 -> Rate Transition67/1
  Rate Transition16/1 -> Mux1/2
  Rate Transition74/1 -> Mux1/59
  Constant34/1 -> Rate Transition35/1
  Rate Transition17/1 -> Mux1/3
  Rate Transition53/1 -> Mux1/38
  Rate Transition39/1 -> Mux1/24
  Rate Transition75/1 -> Mux1/60
  Rate Transition69/1 -> Mux1/54
  Constant54/1 -> Rate Transition55/1
  Rate Transition51/1 -> Mux1/36
  Rate Transition70/1 -> Mux1/55
  Constant41/1 -> Rate Transition42/1
  Constant27/1 -> Rate Transition28/1
  Constant68/1 -> Rate Transition69/1
  Constant47/1 -> Rate Transition48/1
  Constant33/1 -> Rate Transition34/1
  Constant22/1 -> Rate Transition22/1
  Rate Transition32/1 -> Mux1/13
  Constant29/1 -> Rate Transition30/1
  Constant46/1 -> Rate Transition47/1
  Rate Transition24/1 -> Mux1/5
  Rate Transition25/1 -> Mux1/10
  Constant21/1 -> Rate Transition21/1
  Rate Transition45/1 -> Mux1/30
  Rate Transition60/1 -> Mux1/41
  Constant28/1 -> Rate Transition29/1
  Rate Transition61/1 -> Mux1/46
  Rate Transition44/1 -> Mux1/25
  Rate Transition76/1 -> Mux1/57
  Rate Transition72/1 -> Mux1/53
  Rate Transition55/1 -> Mux1/40
  Rate Transition79/1 -> Mux1/63
  Constant67/1 -> Rate Transition68/1
  Constant30/1 -> Rate Transition31/1
  Rate Transition38/1 -> Mux1/23
  Constant55/1 -> Rate Transition56/1
  Rate Transition49/1 -> Mux1/34
  Constant15/1 -> Rate Transition16/1
  Rate Transition67/1 -> Mux1/52
  Constant31/1 -> Rate Transition32/1
  Constant50/1 -> Rate Transition51/1
  Constant89/1 -> Rate Transition94/1
  Rate Transition43/1 -> Mux1/28
  Constant44/1 -> Rate Transition45/1
  Constant51/1 -> Rate Transition52/1
  Constant23/1 -> Rate Transition24/1
  Constant58/1 -> Rate Transition59/1
  Constant45/1 -> Rate Transition46/1
  Constant16/1 -> Rate Transition17/1
  Constant49/1 -> Rate Transition50/1
  Constant52/1 -> Rate Transition53/1
  Constant62/1 -> Rate Transition63/1
  Constant26/1 -> Rate Transition27/1
  Constant25/1 -> Rate Transition26/1
  Constant77/1 -> Rate Transition78/1
  Constant60/1 -> Rate Transition61/1
  Constant63/1 -> Rate Transition64/1
  Constant40/1 -> Rate Transition41/1
  Constant69/1 -> Rate Transition70/1
  Constant53/1 -> Rate Transition54/1
  Constant71/1 -> Rate Transition72/1
  Constant64/1 -> Rate Transition65/1
  Constant65/1 -> Rate Transition66/1
  Rate Transition42/1 -> Mux1/27
  Constant72/1 -> Rate Transition73/1
  Constant76/1 -> Rate Transition77/1
  Rate Transition29/1 -> Mux1/14
  Constant38/1 -> Rate Transition39/1
  Rate Transition19/1 -> Mux1/4
  Rate Transition30/1 -> Mux1/15
  Constant78/1 -> Rate Transition79/1
  Rate Transition21/1 -> Mux1/7
  Rate Transition22/1 -> Mux1/8
  Rate Transition33/1 -> Mux1/18
  Rate Transition20/1 -> Mux1/6
  Constant57/1 -> Rate Transition58/1
  Rate Transition27/1 -> Mux1/12
  Constant79/1 -> Rate Transition80/1
  Constant74/1 -> Rate Transition75/1
  Rate Transition40/1 -> Mux1/21
  Rate Transition46/1 -> Mux1/31
  Rate Transition26/1 -> Mux1/11
  Rate Transition47/1 -> Mux1/32
  Constant73/1 -> Rate Transition74/1
  Rate Transition35/1 -> Mux1/20
  Rate Transition37/1 -> Mux1/22
  Rate Transition31/1 -> Mux1/16
  Rate Transition41/1 -> Mux1/26
  Constant39/1 -> Rate Transition40/1
  Rate Transition57/1 -> Mux1/42
  Rate Transition66/1 -> Mux1/51
  Rate Transition64/1 -> Mux1/45
  Rate Transition56/1 -> Mux1/37
  Rate Transition50/1 -> Mux1/35
  Rate Transition58/1 -> Mux1/43
  Rate Transition65/1 -> Mux1/50
  Rate Transition63/1 -> Mux1/48
  Rate Transition68/1 -> Mux1/49
  Constant59/1 -> Rate Transition60/1

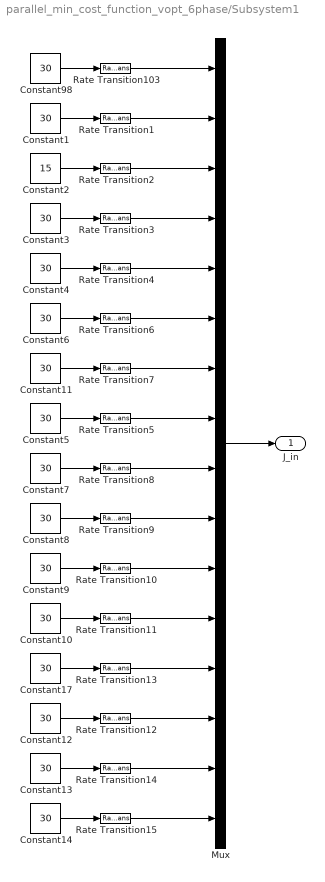
== system parallel_min_cost_function_vopt_6phase/Subsystem1 ==
  Constant{1,3..14,17,98} (15 alike) : Constant  Value=30  OutDataTypeStr=fixdt(1,20,11)  SampleTime=-1
  Constant2 : Constant  Value=15  OutDataTypeStr=fixdt(1,20,11)  SampleTime=-1
  Mux : Mux  Inputs=16
  Rate Transition{1..15,103} (16 alike) : RateTransition  OutPortSampleTime=Rt
  J_in : Outport
  wires:
  Constant1/1 -> Rate Transition1/1
  Rate Transition13/1 -> Mux/13
  Rate Transition103/1 -> Mux/1
  Rate Transition9/1 -> Mux/10
  Rate Transition5/1 -> Mux/8
  Constant11/1 -> Rate Transition7/1
  Rate Transition4/1 -> Mux/5
  Constant12/1 -> Rate Transition12/1
  Rate Transition2/1 -> Mux/3
  Constant3/1 -> Rate Transition3/1
  Rate Transition1/1 -> Mux/2
  Constant5/1 -> Rate Transition5/1
  Constant7/1 -> Rate Transition8/1
  Constant10/1 -> Rate Transition11/1
  Rate Transition7/1 -> Mux/7
  Rate Transition10/1 -> Mux/11
  Rate Transition14/1 -> Mux/15
  Constant4/1 -> Rate Transition4/1
  Rate Transition3/1 -> Mux/4
  Rate Transition8/1 -> Mux/9
  Rate Transition12/1 -> Mux/14
  Constant98/1 -> Rate Transition103/1
  Constant14/1 -> Rate Transition15/1
  Constant2/1 -> Rate Transition2/1
  Constant9/1 -> Rate Transition10/1
  Rate Transition6/1 -> Mux/6
  Constant17/1 -> Rate Transition13/1
  Rate Transition15/1 -> Mux/16
  Constant8/1 -> Rate Transition9/1
  Rate Transition11/1 -> Mux/12
  Constant13/1 -> Rate Transition14/1
  Constant6/1 -> Rate Transition6/1
  Mux/1 -> J_in/1

== matlab function parallel_min_cost_function_vopt_6phase/Min_cost_function_and_vopt/MATLAB Function ==
  data: J_1 input; Index_1 input; J output fixdt(1,20,11); voltages_1 input; J_2 input; Index_2 input; voltages_2 input; J_3 input; Index_3 input; voltages_3 input; J_4 input; Index_4 input; voltages_4 input; J_5 input; Index_5 input; voltages_5 input; J_6 input; Index_6 input; voltages_6 input; J_7 input; Index_7 input; voltages_7 input; J_8 input; Index_8 input; voltages_8 input; J_9 input; Index_9 input; voltages_9 input; J_10 input; Index_10 input; voltages_10 input; J_11 input; Index_11 input; voltages_11 input; J_12 input; Index_12 input; voltages_12 input; J_13 input; Index_13 input; voltages_13 input; J_14 input; Index_14 input; voltages_14 input; J_15 input; Index_15 input; voltages_15 input; J_16 input; Index_16 input; voltages_16 input; Index output int32; min input fixdt(1,20,11); J_default input; voltages output; voltages_default input
function [J, Index, voltages] = fcn(J_1, Index_1, voltages_1, J_2, Index_2, voltages_2, J_3, Index_3, voltages_3, J_4, Index_4, voltages_4, J_5, Index_5, voltages_5, J_6, Index_6, voltages_6, ...
                                    J_7, Index_7, voltages_7, J_8, Index_8, voltages_8, J_9, Index_9, voltages_9, J_10, Index_10, voltages_10, J_11, Index_11, voltages_11, J_12, Index_12, voltages_12, ...
                                    J_13, Index_13, voltages_13, J_14, Index_14, voltages_14, J_15, Index_15, voltages_15, J_16, Index_16, voltages_16, min, J_default,voltages_default)



if J_1 == min
    Index = Index_1;
    voltages = voltages_1;
    J = J_1;
elseif J_2 == min
    Index = Index_2;
    voltages = voltages_2;
    J = J_2;
elseif J_3 == min
    Index = Index_3;
    voltages = voltages_3;
    J = J_3;
elseif J_4 == min
    Index = Index_4;
    voltages = voltages_4;
    J = J_4;
elseif J_5 == min
    Index = Index_5;
    voltages = voltages_5;
    J = J_5;
elseif J_6 == min
    Index = Index_6;
    voltages = voltages_6;
    J = J_6;
elseif J_7 == min
    Index = Index_7;
    voltages = voltages_7;
    J = J_7;
elseif J_8 == min
    Index = Index_8;
    voltages = voltages_8;
    J = J_8;
elseif J_9 == min
    Index = Index_9;
    voltages = voltages_9;
    J = J_9;
elseif J_10 == min
    Index = Index_10;
    voltages = voltages_10;
    J = J_10;
elseif J_11 == min
    Index = Index_11;
    voltages = voltages_11;
    J = J_11;
elseif J_12 == min
    Index = Index_12;
    voltages = voltages_12;
    J = J_12;
elseif J_13 == min
    Index = Index_13;
    voltages = voltages_13;
    J = J_13;
elseif J_14 == min
    Index = Index_14;
    voltages = voltages_14;
    J = J_14;
elseif J_15 == min
    Index = Index_15;
    voltages = voltages_15;
    J = J_15;
elseif J_16 == min
    Index = Index_16;
    voltages = voltages_16;
    J = J_16;
else 
    Index = int32(0);
    J = J_default;
    voltages = voltages_default;
end
